simulink model "sampleModel1729"  (R2023a)
settings: Solver=VariableStepAuto  StartTime=0.0  StopTime=10.0  RelTol=1e-3
libraries: hdlsllib x7, simulink x2
settings Model: Creator=user1  LastModifiedBy=user1

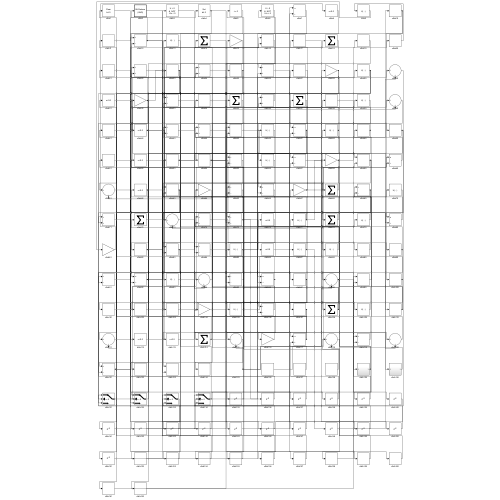
[thumbnail: Simulink's stored preview of the top-level diagram]
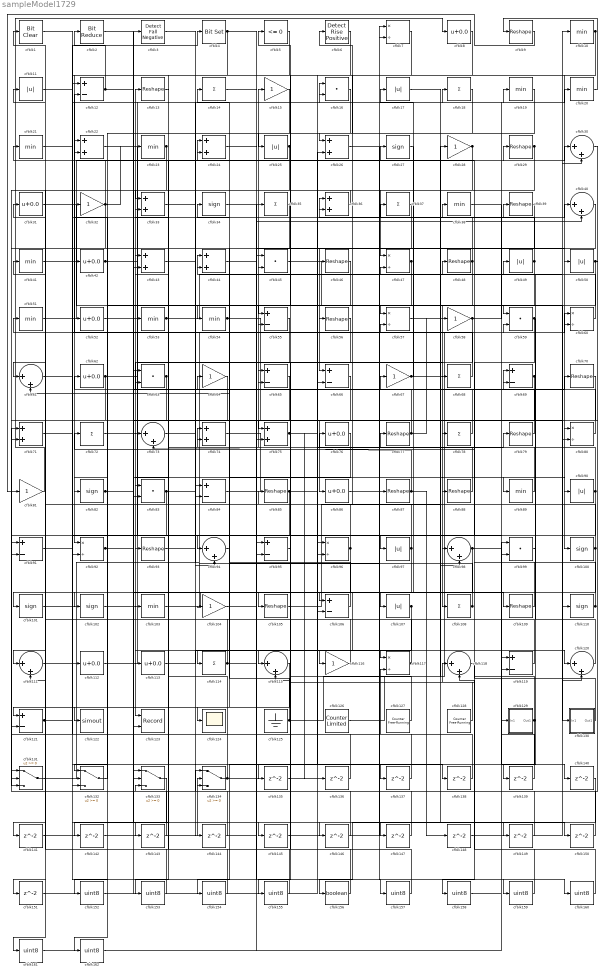
== system sampleModel1729 ==
  cfblk1 : simulink/Logic and Bit Operations/Bit Clear  iBit=0
      settings: LibrarySourceBlock=|
      | hdlsllib/Logic and Bit
      | Operations/Bit Clear
  cfblk{10,19..21,23,38,41,51,53..54,89,103} (12 alike) : MinMax
  cfblk{27,34,82,100..102,110} (7 alike) : Signum
  cfblk{15,28,32,58,64,67,81,104,116} (9 alike) : Gain
  cfblk{9,13,29,39,46,48,56,70,77,79,85,87..88,93,105,109} (16 alike) : Reshape
  cfblk{12,55,65..66,69,84,91,95,106,119,121} (11 alike) : Sum  Inputs=+-
  cfblk{11,17,25,49..50,90,97,107} (8 alike) : Abs  SaturateOnIntegerOverflow=off
  cfblk{14,18,35,37,68,72,78,108,114} (9 alike) : Sum  Inputs=+
  cfblk{30,40,61,73,94,98,111,115,118,120} (10 alike) : Sum  Inputs=|++
  cfblk{8,31,42,52,62,76,86,112..113} (9 alike) : Bias  Bias=0.0  SaturateOnIntegerOverflow=off
  cfblk{7,47,57,60,80,92,96,117} (8 alike) : Product  Inputs=*/  RndMeth=Zero  SaturateOnIntegerOverflow=on
  cfblk122 : ToWorkspace  VariableName=simout  SaveFormat=Timeseries  SampleTime=-1
  cfblk123 : Record  FileSettingsInternal="{\"entries\":[{\"content\":{\"excelSettings\":{\"content\":{},\"type\":\"Streamout.ExcelSettings\"}},\"type\":\"Streamout.FileSettingStorage\",\"uuid\":\"\"}],\"packageUris\":[\"http:\\/\\/schema.mathworks.com\\/mf0\\/streamout_blocks\\/R2020a\"],\"version\":\"1.0\"}"  Layout=[1 1]  SignalsInternal="{\"entries\":[{\"content\":{\"signals\":[{\"content\":{\"blockPath\":[],\"dimensions\":[1],\"domain\":\"\",\"lineColor\":\"#a2142f\",\"plots\":[1],\"port\":1,\"signalID\":3441,\"signalName\":\"XY Graph:1\"},\"type\":\"RecordBlkView.Signal\",\"uuid\":\"\"},{\"content\":{\"blockPath\":[],\"dimensions\":[1],\"domain\":\"\",\"lineColor\":\"#139fff\",\"plots\":[1],\"port\":2,\"signalID\":3444,\"signalName\":\"XY Graph:2\"},\"type\":\"RecordBlkView.Signal\",\"uuid\":\"\"}]},\"type\":\"RecordBlkView.InputSignals\",\"uuid\":\"\"}],\"packageUris\":[\"http:\\/\\/schema.mathworks.com\\/mf0\\/streamout_blocks\\/R2020a\"],\"version\":\"1.0\"}"  VisualizationBindings="{\"xyplotplugin\":{\"info\":[{\"series\":[{\"bindingParametersList\":[{\"parameter\":\"X-Axis\",\"signalID\":3441,\"signalName\":\"XY Graph:1\"},{\"parameter\":\"Y-Axis\",\"signalID\":3444,\"signalName\":\"XY Graph:2\"}],\"seriesID\":36505}],\"subplotID\":1}]}}"  CompatibilityTag=XY  st=-1
  cfblk124 : Scope
  cfblk125 : Ground
  cfblk126 : hdlsllib/Sources/Counter Limited  uplimit=7  tsamp=-1
  cfblk127 : hdlsllib/Sources/Counter Free-Running  NumBits=16  tsamp=-1
  cfblk128 : hdlsllib/Sources/Counter Free-Running  NumBits=16  tsamp=-1
  cfblk129 : Subsystem
      settings: LibrarySourceBlock=|
      | hdlsllib/Ports &
      | Subsystems/Subsystem
  cfblk130 : Subsystem
      settings: LibrarySourceBlock=|
      | hdlsllib/Ports &
      | Subsystems/Subsystem
  cfblk{131..134} (4 alike) : Switch  SaturateOnIntegerOverflow=off  InputSameDT=off
  cfblk{135..151} (17 alike) : Delay  SampleTime=1
  cfblk{152..155,157..162} (10 alike) : DataTypeConversion  OutDataTypeStr=uint8  SaturateOnIntegerOverflow=off  RndMeth=Floor
  cfblk156 : DataTypeConversion  OutDataTypeStr=boolean  SaturateOnIntegerOverflow=off  RndMeth=Floor
  cfblk{16,45,59,63,83,99} (6 alike) : DotProduct  OutDataTypeStr=Inherit: Inherit via internal rule
  cfblk2 : hdlsllib/Logic and Bit Operations/Bit Reduce  mode=AND
  cfblk{22,24,26,33,36,43..44,71,74..75} (10 alike) : Sum
  cfblk3 : hdlsllib/Logic and Bit Operations/Detect Fall Negative  vinit=0  OutDataTypeStr=boolean
  cfblk4 : simulink/Logic and Bit Operations/Bit Set  iBit=0
      settings: LibrarySourceBlock=|
      | hdlsllib/Logic and Bit
      | Operations/Bit Set
  cfblk5 : hdlsllib/Logic and Bit Operations/Compare To Zero  relop=<=  OutDataTypeStr=boolean
  cfblk6 : hdlsllib/Logic and Bit Operations/Detect Rise Positive  vinit=0  OutDataTypeStr=boolean
  wires:
  cfblk72/1 -> cfblk27/1
  cfblk5/1 -> cfblk92/1
  cfblk66/1 -> cfblk86/1
  cfblk10/1 -> cfblk100/1, cfblk26/1
  cfblk85/1 -> cfblk30/1, cfblk79/1, cfblk121/2
  cfblk88/1 -> cfblk15/1
  cfblk47/1 -> cfblk66/1, cfblk82/1
  cfblk101/1 -> cfblk60/1
  cfblk51/1 -> cfblk38/1
  cfblk110/1 -> cfblk44/1, cfblk69/2
  cfblk69/1 -> cfblk123/1, cfblk96/2
  cfblk126/1 -> cfblk60/2
  cfblk33/1 -> cfblk84/1
  cfblk64/1 -> cfblk92/2
  cfblk31/1 -> cfblk59/1
  cfblk91/1 -> cfblk97/1
  cfblk81/1 -> cfblk8/1
  cfblk75/1 -> cfblk136/1, cfblk137/1
  cfblk23/1 -> cfblk123/2, cfblk162/1
  cfblk79/1 -> cfblk64/1
  cfblk39/1 -> cfblk94/1
  cfblk53/1 -> cfblk10/1, cfblk57/1
  cfblk80/1 -> cfblk13/1
  cfblk105/1 -> cfblk28/1
  cfblk27/1 -> cfblk107/1
  cfblk70/1 -> cfblk84/2
  cfblk83/1 -> cfblk91/2, cfblk40/1
  cfblk120/1 -> cfblk49/1
  cfblk82/1 -> cfblk70/1, cfblk146/1
  cfblk65/1 -> cfblk101/1
  cfblk38/1 -> cfblk129/1(In1)
  cfblk62/1 -> cfblk19/1, cfblk121/1
  cfblk132/1 -> cfblk62/1
  cfblk6/1 -> cfblk66/2
  cfblk84/1 -> cfblk89/1
  cfblk50/1 -> cfblk80/1, cfblk142/1
  cfblk48/1 -> cfblk108/1, cfblk36/1
  cfblk59/1 -> cfblk98/1, cfblk139/1
  cfblk131/1 -> cfblk3/1
  cfblk121/1 -> cfblk16/2, cfblk145/1
  cfblk112/1 -> cfblk16/1
  cfblk103/1 -> cfblk7/2
  cfblk114/1 -> cfblk41/1, cfblk40/2
  cfblk56/1 -> cfblk93/1
  cfblk52/1 -> cfblk119/2
  cfblk92/1 -> cfblk39/1, cfblk57/2
  cfblk102/1 -> cfblk67/1
  cfblk42/1 -> cfblk94/2, cfblk102/1, cfblk87/1
  cfblk107/1 -> cfblk104/1, cfblk113/1
  cfblk43/1 -> cfblk18/1
  cfblk37/1 -> cfblk56/1
  cfblk76/1 -> cfblk114/1
  cfblk20/1 -> cfblk9/1
  cfblk14/1 -> cfblk50/1
  cfblk12/1 -> cfblk106/1, cfblk75/2, cfblk2/1
  cfblk11/1 -> cfblk4/1
  cfblk125/1 -> cfblk44/2, cfblk29/1, cfblk98/2
  cfblk60/1 -> cfblk17/1
  cfblk63/1 -> cfblk71/2, cfblk151/1
  cfblk109/1 -> cfblk72/1
  cfblk55/1 -> cfblk103/1
  cfblk22/1 -> cfblk78/1
  cfblk89/1 -> cfblk21/1
  cfblk9/1 -> cfblk81/1
  cfblk67/1 -> cfblk59/2, cfblk47/2
  cfblk46/1 -> cfblk54/1
  cfblk36/1 -> cfblk33/1
  cfblk94/1 -> cfblk34/1
  cfblk16/1 -> cfblk83/1
  cfblk68/1 -> cfblk12/2
  cfblk78/1 -> cfblk43/1
  cfblk21/1 -> cfblk112/1
  cfblk49/1 -> cfblk106/2, cfblk36/2
  cfblk40/1 -> cfblk73/1
  cfblk77/1 -> cfblk75/1, cfblk58/1, cfblk32/1
  cfblk97/1 -> cfblk111/1, cfblk116/1, cfblk14/1
  cfblk25/1 -> cfblk61/1, cfblk131/3
  cfblk58/1 -> cfblk20/1, cfblk115/2
  cfblk54/1 -> cfblk110/1, cfblk48/1, cfblk80/2
  cfblk117/1 -> cfblk85/1, cfblk24/2
  cfblk108/1 -> cfblk65/1, cfblk74/2
  cfblk134/1 -> cfblk63/2, cfblk26/2
  cfblk45/1 -> cfblk130/1(In1)
  cfblk113/1 -> cfblk120/1
  cfblk95/1 -> cfblk65/2
  cfblk128/1 -> cfblk5/1
  cfblk74/1 -> cfblk96/1
  cfblk106/1 -> cfblk61/2
  cfblk28/1 -> cfblk47/1, cfblk42/1
  cfblk130/1(Out1) -> cfblk22/1
  cfblk96/1 -> cfblk124/1, cfblk11/1
  cfblk2/1 -> cfblk88/1
  cfblk116/1 -> cfblk52/1
  cfblk4/1 -> cfblk120/2, cfblk132/3
  cfblk111/1 -> cfblk37/1
  cfblk90/1 -> cfblk6/1, cfblk105/1
  cfblk7/1 -> cfblk25/1
  cfblk100/1 -> cfblk76/1, cfblk155/1
  cfblk127/1 -> cfblk51/1
  cfblk32/1 -> cfblk131/2, cfblk22/2, cfblk23/1, cfblk132/1
  cfblk3/1 -> cfblk117/1
  cfblk18/1 -> cfblk55/1
  cfblk29/1 -> cfblk111/2, cfblk83/2, cfblk132/2
  cfblk87/1 -> cfblk73/2, cfblk148/1
  cfblk71/1 -> cfblk53/1
  cfblk24/1 -> cfblk68/1
  cfblk30/1 -> cfblk134/2
  cfblk19/1 -> cfblk122/1
  cfblk99/1 -> cfblk69/1
  cfblk15/1 -> cfblk95/2
  cfblk41/1 -> cfblk24/1
  cfblk17/1 -> cfblk90/1
  cfblk98/1 -> cfblk115/1, cfblk140/1
  cfblk44/1 -> cfblk109/1
  cfblk119/1 -> cfblk31/1
  cfblk129/1(Out1) -> cfblk74/1, cfblk77/1, cfblk154/1
  cfblk61/1 -> cfblk135/1
  cfblk135/1 -> cfblk55/2
  cfblk136/1 -> cfblk12/1
  cfblk137/1 -> cfblk117/2
  cfblk93/1 -> cfblk138/1
  cfblk138/1 -> cfblk91/1
  cfblk139/1 -> cfblk119/1
  cfblk115/1 -> cfblk141/1
  cfblk141/1 -> cfblk134/3
  cfblk142/1 -> cfblk95/1
  cfblk13/1 -> cfblk143/1
  cfblk143/1 -> cfblk63/1
  cfblk73/1 -> cfblk144/1
  cfblk144/1 -> cfblk33/2
  cfblk145/1 -> cfblk7/1
  cfblk146/1 -> cfblk134/1
  cfblk34/1 -> cfblk147/1
  cfblk147/1 -> cfblk131/1
  cfblk148/1 -> cfblk30/2
  cfblk26/1 -> cfblk149/1
  cfblk149/1 -> cfblk71/1
  cfblk57/1 -> cfblk150/1
  cfblk150/1 -> cfblk45/1
  cfblk151/1 -> cfblk43/2
  cfblk133/1 -> cfblk152/1
  cfblk152/1 -> cfblk46/1
  cfblk8/1 -> cfblk153/1
  cfblk153/1 -> cfblk133/1
  cfblk154/1 -> cfblk133/2
  cfblk155/1 -> cfblk133/3
  cfblk140/1 -> cfblk156/1
  cfblk156/1 -> cfblk1/1
  cfblk1/1 -> cfblk157/1
  cfblk157/1 -> cfblk45/2
  cfblk118/1 -> cfblk158/1
  cfblk158/1 -> cfblk99/1
  cfblk104/1 -> cfblk159/1
  cfblk159/1 -> cfblk118/1
  cfblk86/1 -> cfblk160/1
  cfblk160/1 -> cfblk118/2
  cfblk35/1 -> cfblk161/1
  cfblk161/1 -> cfblk99/2
  cfblk162/1 -> cfblk35/1

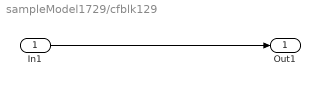
== system sampleModel1729/cfblk129 ==
  In1 : Inport
  Out1 : Outport
  wires:
  In1/1 -> Out1/1

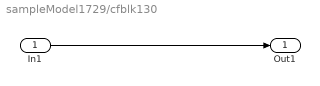
== system sampleModel1729/cfblk130 ==
  In1 : Inport
  Out1 : Outport
  wires:
  In1/1 -> Out1/1
